simulink model "nichtlinearesModell"  (R2016b)
settings: Solver=VariableStepAuto  StartTime=0.0  StopTime=30  RelTol=1e-3
values from neighbouring files (symbols this model uses):
  Ak = [A1                      E*C_s ... (first row only)    [StartSim.m]
  B1 = [0 b2 0 b4]'    [RiccatiBerechnung_Anlage.m]    (also in RiccatiBerechnunguPlot_Simulation.m; StartSim.m)
  Bk = [B1; zeros(1,size(B1,2))]    [StartSim.m]
  Ck = [C1 zeros(size(C1,1),1)]    [StartSim.m]
  K1 = 1    [RiccatiBerechnung_Anlage.m]    (also in RiccatiBerechnunguPlot_Simulation.m; StartSim.m)
  K2 = 1    [RiccatiBerechnung_Anlage.m]    (also in RiccatiBerechnunguPlot_Simulation.m; StartSim.m)
  L_0 = 0.5    [RiccatiBerechnunguPlot_Simulation.m]    (also in StartSim.m = 0.6)
  phi_0 = 0    [RiccatiBerechnunguPlot_Simulation.m]    (also in StartSim.m)
  r1 = 0.0191    [LQG.m]    (also in RiccatiBerechnung_Anlage.m = 0.046; RiccatiBerechnunguPlot_Simulation.m = 0.046; StartSim.m = 0.046)
  r2 = 0.015915    [LQG.m]    (also in RiccatiBerechnung_Anlage.m = 0.021975; RiccatiBerechnunguPlot_Simulation.m = 0.021975; StartSim.m = 0.025)
  T1 = 0.1    [LQG.m]    (also in RiccatiBerechnung_Anlage.m = 0.03032; RiccatiBerechnunguPlot_Simulation.m = 0.03032; StartSim.m = 0.03032)
  T2 = 0.1    [LQG.m]    (also in RiccatiBerechnung_Anlage.m = 0.0247; RiccatiBerechnunguPlot_Simulation.m = 0.0247; StartSim.m = 0.03032)
  ue1 = 6    [RiccatiBerechnung_Anlage.m]    (also in RiccatiBerechnunguPlot_Simulation.m; StartSim.m)
  ue2 = 3    [RiccatiBerechnung_Anlage.m]    (also in RiccatiBerechnunguPlot_Simulation.m; StartSim.m)
  x_0 = 2.54    [RiccatiBerechnunguPlot_Simulation.m]    (also in StartSim.m = 1.3)
undefined symbols (not defined in the file or in its folder): Continuous, K, Time
libraries: simulink_extras x3, simulink x2, ctrlSharedLib x1
settings Model: Creator=Patrick  LastModifiedBy=Patrick

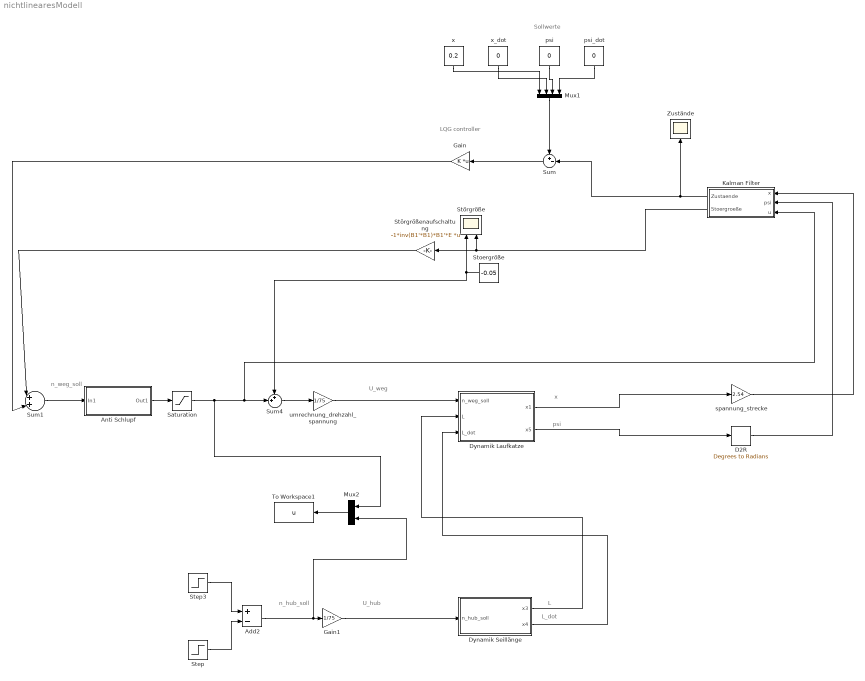
== system nichtlinearesModell ==
  note: n_hub_soll
  note: U_hub
  note: L
  note: L_dot
  note: x
  note: psi
  note: LQG controller
  note: U_weg
  note: n_weg_soll
  note: Sollwerte
  Add2 : Sum  Inputs=+-
  Anti Schlupf : Subsystem
  D2R : simulink_extras/Transformations/Degrees to Radians
  Dynamik Laufkatze : Subsystem
  Dynamik Seillänge : Subsystem
  Gain : Gain  Gain=K  Multiplication=Matrix(K*u)
  Gain1 : Gain  Gain=1/75
  Kalman Filter : Subsystem
  Mux1 : Mux
  Mux2 : Mux  Inputs=2
  Saturation : Saturate  UpperLimit=75  LowerLimit=-75
  Step : Step  Time=0  After=0  SampleTime=0
  Step3 : Step  Time=0  After=0  SampleTime=0
  Stoergröße : Constant  Value=-0.05
  Störgröße : Scope  NumInputPorts=2
  Störgrößenaufschaltung : Gain  Gain=-1*inv(B1'*B1)*B1'*E  Multiplication=Matrix(K*u)
  Sum : Sum  Inputs=+-|
  Sum1 : Sum  Inputs=|++|
  Sum4 : Sum  Inputs=++|
  To Workspace1 : ToWorkspace  VariableName=u  SampleTime=-1
  Zustände : Scope
  psi : Constant  Value=0
  psi_dot : Constant  Value=0
  spannung_strecke : Gain  Gain=2.54
  umrechnung_drehzahl_spannung : Gain  Gain=1/75
  x : Constant  Value=0.2
  x_dot : Constant  Value=0
  wires:
  Add2/1 -> Mux2/2, Gain1/1
  Gain1/1 -> Dynamik Seillänge/1(n_hub_soll)
  Step3/1 -> Add2/1
  Dynamik Seillänge/1(x3) -> Dynamik Laufkatze/2(L)
  Step/1 -> Add2/2
  Dynamik Seillänge/2(x4) -> Dynamik Laufkatze/3(L_dot)
  Mux2/1 -> To Workspace1/1
  Sum/1 -> Gain/1
  Gain/1 -> Sum1/2
  Dynamik Laufkatze/1(x1) -> spannung_strecke/1
  Kalman Filter/1(Zustaende) -> Zustände/1, Sum/2
  Stoergröße/1 -> Sum4/1, Störgröße/1
  umrechnung_drehzahl_spannung/1 -> Dynamik Laufkatze/1(n_weg_soll)
  Anti Schlupf/1(Out1) -> Saturation/1
  Kalman Filter/2(Stoergroeße) -> Störgröße/2, Störgrößenaufschaltung/1
  Sum1/1 -> Anti Schlupf/1(In1)
  spannung_strecke/1 -> Kalman Filter/1(x)
  D2R/1 -> Kalman Filter/2(psi)
  Saturation/1 -> Mux2/1, Kalman Filter/3(u), Sum4/2
  Mux1/1 -> Sum/1
  psi_dot/1 -> Mux1/4
  x_dot/1 -> Mux1/2
  psi/1 -> Mux1/3
  x/1 -> Mux1/1
  Sum4/1 -> umrechnung_drehzahl_spannung/1
  Störgrößenaufschaltung/1 -> Sum1/1
  Dynamik Laufkatze/2(x5) -> D2R/1

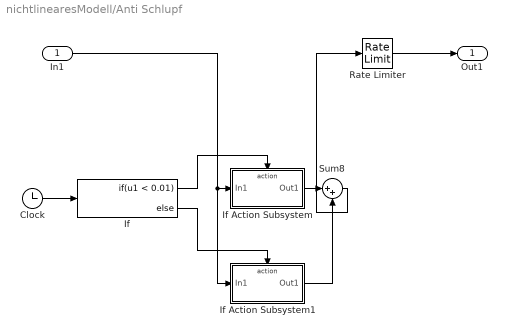
== system nichtlinearesModell/Anti Schlupf ==
  In1 : Inport
  Clock : Clock
  If : If  IfExpression=u1 < 0.01
  If Action Subsystem : Subsystem  TreatAsAtomicUnit=on
  If Action Subsystem1 : Subsystem  TreatAsAtomicUnit=on
  Rate Limiter : RateLimiter  RisingSlewLimit=9.57  FallingSlewLimit=-9.57  SampleTimeMode=inherited
  Sum8 : Sum  Inputs=|++
  Out1 : Outport
  wires:
  In1/1 -> If Action Subsystem1/1(In1), If Action Subsystem/1(In1)
  If Action Subsystem/1(Out1) -> Sum8/1
  If Action Subsystem1/1(Out1) -> Sum8/2
  Sum8/1 -> Rate Limiter/1
  If/1 -> If Action Subsystem/Action
  If/2 -> If Action Subsystem1/Action
  Rate Limiter/1 -> Out1/1
  Clock/1 -> If/1

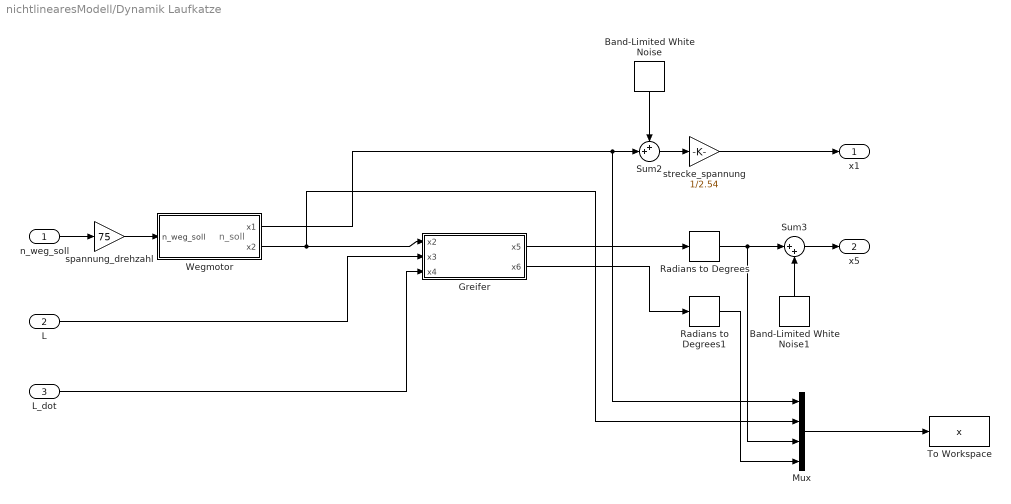
== system nichtlinearesModell/Dynamik Laufkatze ==
  note: n_soll
  n_weg_soll : Inport
  L : Inport  Port=2
  L_dot : Inport  Port=3
  Band-Limited White Noise : simulink/Sources/Band-Limited White Noise  Cov=0.00000001  Ts=0.001  seed=[23341]
  Band-Limited White Noise1 : simulink/Sources/Band-Limited White Noise  Cov=0.0000001  Ts=0.001  seed=[23341]
  Greifer : Subsystem
  Mux : Mux
  Radians to Degrees : simulink_extras/Transformations/Radians to Degrees
  Radians to Degrees1 : simulink_extras/Transformations/Radians to Degrees
  Sum2 : Sum  Inputs=++|
  Sum3 : Sum  Inputs=|++
  To Workspace : ToWorkspace  VariableName=x  SampleTime=-1
  Wegmotor : Subsystem
  spannung_drehzahl : Gain  Gain=75
  strecke_spannung : Gain  Gain=1/2.54
  x1 : Outport
  x5 : Outport  Port=2
  wires:
  n_weg_soll/1 -> spannung_drehzahl/1
  Wegmotor/1(x1) -> Sum2/2, Mux/1
  Wegmotor/2(x2) -> Mux/2, Greifer/1(x2)
  Greifer/1(x5) -> Radians to Degrees/1
  Greifer/2(x6) -> Radians to Degrees1/1
  L/1 -> Greifer/2(x3)
  L_dot/1 -> Greifer/3(x4)
  spannung_drehzahl/1 -> Wegmotor/1(n_weg_soll)
  Radians to Degrees1/1 -> Mux/4
  Mux/1 -> To Workspace/1
  Radians to Degrees/1 -> Sum3/1, Mux/3
  strecke_spannung/1 -> x1/1
  Band-Limited White Noise1/1 -> Sum3/2
  Sum3/1 -> x5/1
  Sum2/1 -> strecke_spannung/1
  Band-Limited White Noise/1 -> Sum2/1

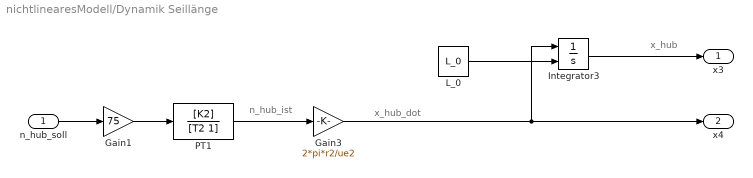
== system nichtlinearesModell/Dynamik Seillänge ==
  note: n_hub_ist
  note: x_hub_dot
  note: x_hub
  n_hub_soll : Inport
  Gain1 : Gain  Gain=75
  Gain3 : Gain  Gain=2*pi*r2/ue2
  Integrator3 : Integrator  InitialConditionSource=external
  L_0 : Constant  Value=L_0
  PT1 : TransferFcn  Numerator=[K2]  Denominator=[T2 1]
  x3 : Outport
  x4 : Outport  Port=2
  wires:
  n_hub_soll/1 -> Gain1/1
  PT1/1 -> Gain3/1
  Integrator3/1 -> x3/1
  L_0/1 -> Integrator3/2
  Gain3/1 -> Integrator3/1, x4/1
  Gain1/1 -> PT1/1

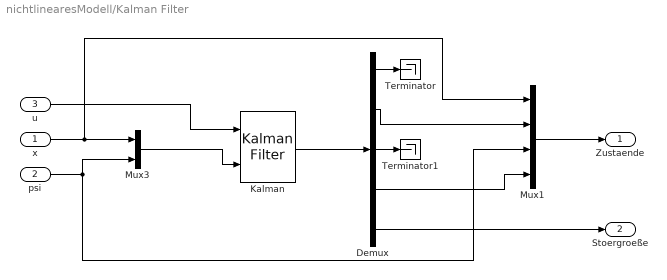
== system nichtlinearesModell/Kalman Filter ==
  x : Inport
  psi : Inport  Port=2
  u : Inport  Port=3
  Demux : Demux  Outputs=5
  Kalman : ctrlSharedLib/Kalman Filter  TimeDomain=Continuous-Time  UseCurrentEstimator=on  ModelSource=Individual A, B, C, D matrices  ModelSourceVariable=ss(Ak,Bk,Ck,0)  A=Ak  B=Bk  C=Ck  D=0  NumberOfStates=1  NumberOfInputs=1  NumberOfOutputs=1  InitialEstimateSource=Dialog  X0=0  P0=10  UseK=off  UseGH=off  NumberOfProcessNoiseInputs=1  G=Bk  TimeInvariantG=on  H=0  TimeInvariantH=on  Q=1  TimeInvariantQ=on  R=45  TimeInvariantR=on  N=0  TimeInvariantN=on  AddInputPort=on  AddEnablePort=off  ExternalReset=none  OutputEstimatedY=off  OutputP=off  Ts=-1
  Mux1 : Mux
  Mux3 : Mux  Inputs=2
  Terminator : Terminator
  Terminator1 : Terminator
  Zustaende : Outport
  Stoergroeße : Outport  Port=2
  wires:
  Mux3/1 -> Kalman/2
  Kalman/1 -> Demux/1
  psi/1 -> Mux1/3, Mux3/2
  x/1 -> Mux1/1, Mux3/1
  u/1 -> Kalman/1
  Demux/2 -> Mux1/2
  Demux/4 -> Mux1/4
  Mux1/1 -> Zustaende/1
  Demux/5 -> Stoergroeße/1
  Demux/1 -> Terminator/1
  Demux/3 -> Terminator1/1

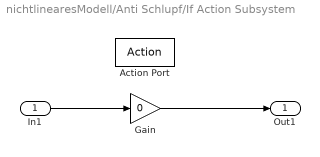
== system nichtlinearesModell/Anti Schlupf/If Action Subsystem ==
  In1 : Inport
  Action Port : ActionPort  ActionType=then
  Gain : Gain  Gain=0
  Out1 : Outport
  wires:
  In1/1 -> Gain/1
  Gain/1 -> Out1/1

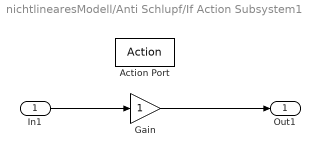
== system nichtlinearesModell/Anti Schlupf/If Action Subsystem1 ==
  In1 : Inport
  Action Port : ActionPort  ActionType=else
  Gain : Gain
  Out1 : Outport
  wires:
  In1/1 -> Gain/1
  Gain/1 -> Out1/1

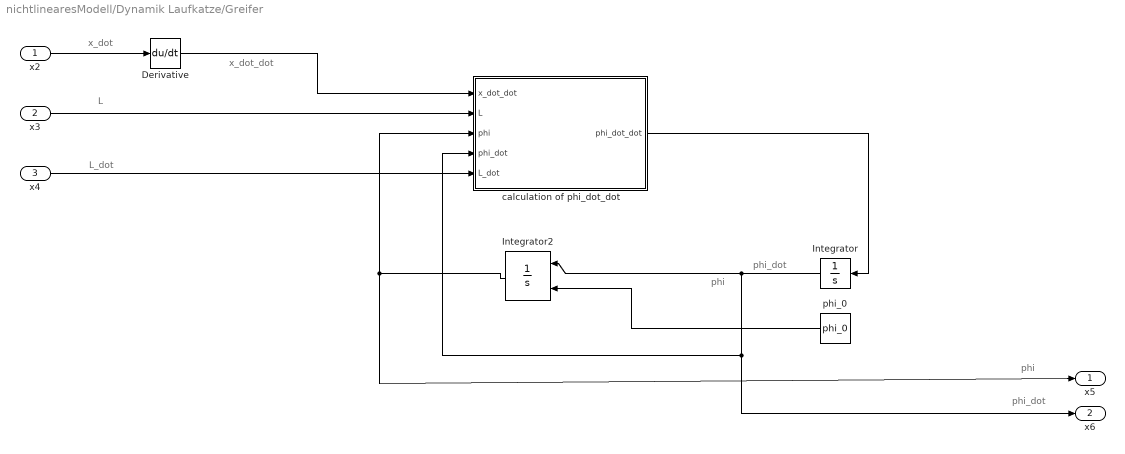
== system nichtlinearesModell/Dynamik Laufkatze/Greifer ==
  note: phi
  note: phi
  note: x_dot
  note: L
  note: phi_dot
  note: phi_dot
  note: x_dot_dot
  note: L_dot
  x2 : Inport
  x3 : Inport  Port=2
  x4 : Inport  Port=3
  Derivative : Derivative
  Integrator : Integrator
  Integrator2 : Integrator  InitialConditionSource=external
  calculation of phi_dot_dot : MATLAB Function  TreatAsAtomicUnit=on
  phi_0 : Constant  Value=phi_0
  x5 : Outport
  x6 : Outport  Port=2
  wires:
  Derivative/1 -> calculation of phi_dot_dot/1(x_dot_dot)
  x2/1 -> Derivative/1
  Integrator/1 -> x6/1, calculation of phi_dot_dot/4(phi_dot), Integrator2/1
  x3/1 -> calculation of phi_dot_dot/2(L)
  calculation of phi_dot_dot/1(phi_dot_dot) -> Integrator/1
  Integrator2/1 -> x5/1, calculation of phi_dot_dot/3(phi)
  x4/1 -> calculation of phi_dot_dot/5(L_dot)
  phi_0/1 -> Integrator2/2

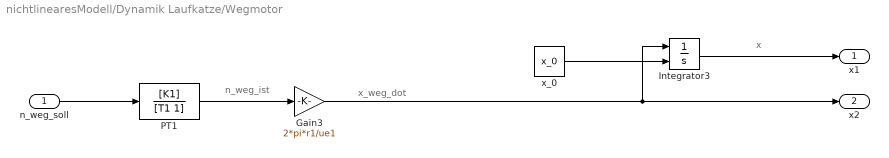
== system nichtlinearesModell/Dynamik Laufkatze/Wegmotor ==
  note: n_weg_ist
  note: x
  note: x_weg_dot
  n_weg_soll : Inport
  Gain3 : Gain  Gain=2*pi*r1/ue1
  Integrator3 : Integrator  InitialConditionSource=external
  PT1 : TransferFcn  Numerator=[K1]  Denominator=[T1 1]
  x_0 : Constant  Value=x_0
  x1 : Outport
  x2 : Outport  Port=2
  wires:
  x_0/1 -> Integrator3/2
  n_weg_soll/1 -> PT1/1
  PT1/1 -> Gain3/1
  Integrator3/1 -> x1/1
  Gain3/1 -> Integrator3/1, x2/1

== matlab function nichtlinearesModell/Dynamik Laufkatze/Greifer/calculation of phi_dot_dot ==
  data: x_dot_dot input; phi_dot_dot output; L input; phi input; phi_dot input; L_dot input
function phi_dot_dot = fcn(x_dot_dot,L,phi,phi_dot,L_dot)

phi_dot_dot = -(cos(phi)/L)*x_dot_dot-9.81/L*sin(phi)-2*L_dot*phi_dot;
